simulink model "inverse_kinematics"  (R2025b)
settings: Solver=VariableStepAuto  StartTime=0.0  StopTime=10.0  FixedStep=0.001  RelTol=1e-3
undefined symbols (not defined in the file or in its folder): Levenberg, Marquardt
libraries: robotcorelib x2, robotmaniplib x2, SignalEditorBlockLib x2
settings Model: Creator=niran  LastModifiedBy=rowan
settings OptimizationCC: OptimizeBlockIOStorage=off  ZeroExternalMemoryAtStartup=off  ZeroInternalMemoryAtStartup=off  OptimizeDataStoreBuffers=off  BusAssignmentInplaceUpdate=off
settings DebuggingCC: SFUnexpectedBacktrackingDiag=warning  SFNoUnconditionalDefaultTransitionDiag=warning
settings RTWCC: GenCodeOnly=on  GenerateReport=on  BuildConfiguration=Debug  LaunchReport=on  TargetLang=C++
settings CodeAppCC: ForceParamTrailComments=on  MATLABSourceComments=on  EnableCustomComments=on
settings GRTTargetCC: MultiInstanceErrorCode=Warning  TargetLangStandard=C++11 (ISO)  CombineSignalStateStructs=on  CodeInterfacePackaging=C++ class  SupportVariableSizeSignals=on

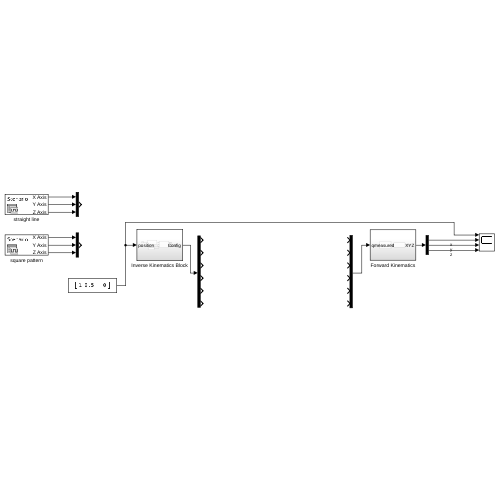
[thumbnail: Simulink's stored preview of the top-level diagram]
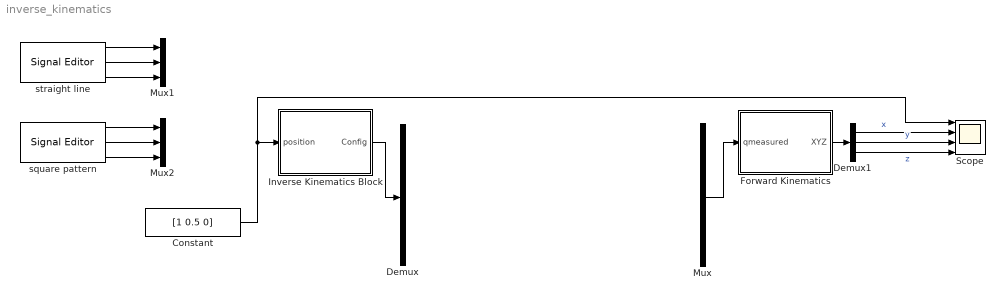
== system inverse_kinematics ==
  Constant : Constant  Value=[1 0.5 0]
  Demux : Demux  Outputs=6
  Demux1 : Demux  Outputs=3
  Forward Kinematics : Subsystem
  Inverse Kinematics Block : Subsystem
  Mux : Mux  Inputs=6
  Mux1 : Mux  Inputs=3
  Mux2 : Mux  Inputs=3
  Scope : Scope  NumInputPorts=4
      settings: ActiveDisplayYMinimum=-0.3  ActiveDisplayYMaximum=0.7
  square pattern : SignalEditorBlockLib/Signal Editor  FileName=signal_editor.mat  ActiveScenario=Scenario  ActiveSignal=X Axis  IsBus=off  OutputBusObjectStr=Bus: BusObject  SampleTime=0.001  ZeroCross=off  OutputAfterFinalValue=Holding final value  Unit=inherit  PreserveSignalName=on  ApplySigPropsToAllScenarios=on  ApplySigPropsToAllSignals=off  SignalPropertySource=Dialog parameters
  straight line : SignalEditorBlockLib/Signal Editor  FileName=signal_editor_1.mat  ActiveScenario=Scenario  ActiveSignal=X Axis  IsBus=off  OutputBusObjectStr=Bus: BusObject  SampleTime=0.001  ZeroCross=off  OutputAfterFinalValue=Holding final value  Unit=inherit  PreserveSignalName=on  ApplySigPropsToAllScenarios=on  ApplySigPropsToAllSignals=off  SignalPropertySource=Dialog parameters
  wires:
  Forward Kinematics/1(XYZ) -> Demux1/1
  straight line/1 -> Mux1/1
  straight line/2 -> Mux1/2
  Mux/1 -> Forward Kinematics/1(qmeasured)
  Demux1/2 -> Scope/3  "y"
  Demux1/1 -> Scope/2  "x"
  Demux1/3 -> Scope/4  "z"
  square pattern/2 -> Mux2/2
  square pattern/1 -> Mux2/1
  square pattern/3 -> Mux2/3
  Inverse Kinematics Block/1(Config) -> Demux/1
  Constant/1 -> Scope/1, Inverse Kinematics Block/1(position)
  straight line/3 -> Mux1/3

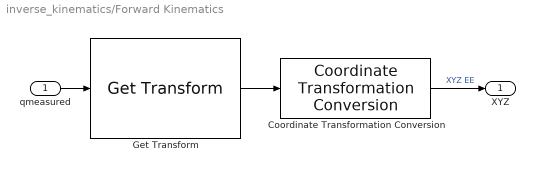
== system inverse_kinematics/Forward Kinematics ==
  qmeasured : Inport
  Coordinate Transformation Conversion : robotcorelib/Coordinate Transformation Conversion  InputRepresentation=Homogeneous Transformation  InputEulerSequence=ZYX  ShowTrVecInputPort=on  OutputRepresentation=Translation Vector  OutputEulerSequence=ZYX  ShowTrVecOutputPort=on  SimulateUsing=Interpreted execution
  Get Transform : robotmaniplib/Get Transform  RigidBodyTree=robotic_arm  SourceBody=Base  TargetBody=Body6  SimulateUsing=Interpreted execution
  XYZ : Outport
  wires:
  Get Transform/1 -> Coordinate Transformation Conversion/1
  Coordinate Transformation Conversion/1 -> XYZ/1  "XYZ EE"
  qmeasured/1 -> Get Transform/1

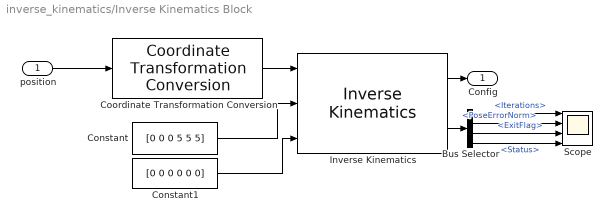
== system inverse_kinematics/Inverse Kinematics Block ==
  position : Inport
  Bus Selector : BusSelector  OutputSignals=Iterations,PoseErrorNorm,ExitFlag,Status
  Constant : Constant  Value=[0 0 0 5 5 5]
  Constant1 : Constant  Value=[0 0 0 0 0 0]
  Coordinate Transformation Conversion : robotcorelib/Coordinate Transformation Conversion  InputRepresentation=Translation Vector  InputEulerSequence=ZYX  ShowTrVecInputPort=on  OutputRepresentation=Homogeneous Transformation  OutputEulerSequence=ZYX  ShowTrVecOutputPort=on  SimulateUsing=Interpreted execution
  Inverse Kinematics : robotmaniplib/Inverse Kinematics  RigidBodyTree=robotic_arm  EndEffector=Body6  ShowInfo=on  SolverName=Levenberg-Marquardt  EnforceJointLimits=on  MaxIterations=1500  MaxTime=10  GradientTolerance=1e-3  SolutionTolerance=1e-2  StepTolerance=1e-14  ConstraintTolerance=1e-6  ErrorChangeTolerance=1e-3  UseErrorDamping=on  DampingBias=0.0025  SimulateUsing=Interpreted execution
  Scope : Scope  NumInputPorts=4
      settings: ActiveDisplayYMinimum=-173.87499999999997  ActiveDisplayYMaximum=1594.875
  Config : Outport
  wires:
  Coordinate Transformation Conversion/1 -> Inverse Kinematics/1
  Inverse Kinematics/1 -> Config/1
  Constant/1 -> Inverse Kinematics/2
  Inverse Kinematics/2 -> Bus Selector/1
  Constant1/1 -> Inverse Kinematics/3
  position/1 -> Coordinate Transformation Conversion/1
  Bus Selector/1 -> Scope/1  "<Iterations>"
  Bus Selector/2 -> Scope/2  "<PoseErrorNorm>"
  Bus Selector/3 -> Scope/3  "<ExitFlag>"
  Bus Selector/4 -> Scope/4  "<Status>"
